simulink model "Adaptive_flux_observer_with_Rs_and_Rr_estimator"  (R2021a)
settings: Solver=FixedStepDiscrete  StartTime=0.0  StopTime=10.0  FixedStep=1e-5  RelTol=1e-3
undefined symbols (not defined in the file): DiscIntNeverNeededParam
settings Model: Creator=Mehra  LastModifiedBy=Mehra

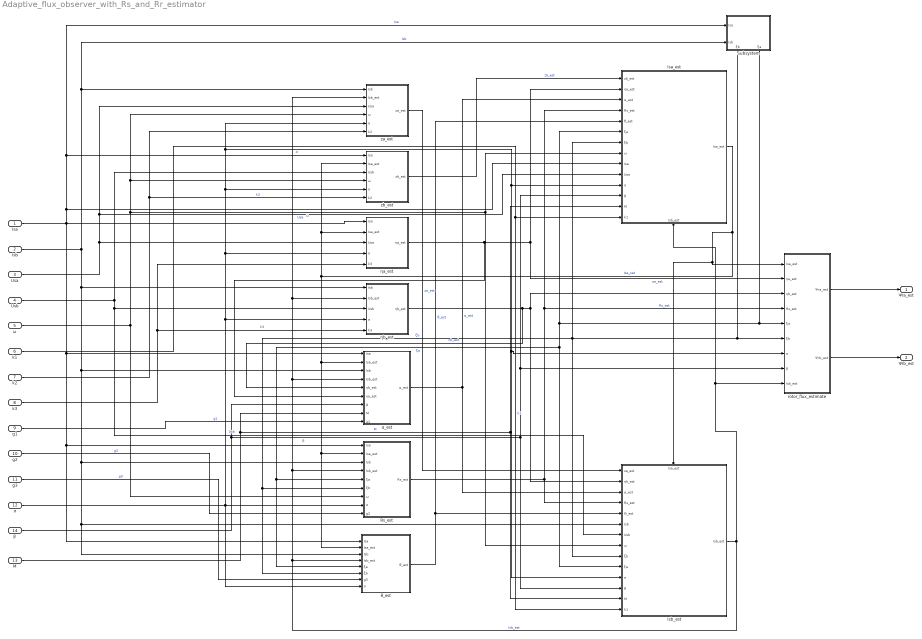
== system Adaptive_flux_observer_with_Rs_and_Rr_estimator ==
  Isa : Inport
  Isb : Inport  Port=2
  Usa : Inport  Port=3
  Usb : Inport  Port=4
  ω : Inport  Port=5
  k1 : Inport  Port=6
  k2 : Inport  Port=7
  k3 : Inport  Port=8
  g1 : Inport  Port=9
  g2 : Inport  Port=10
  g3 : Inport  Port=11
  σ : Inport  Port=12
  M : Inport  Port=13
  β : Inport  Port=14
  Isa_est : Subsystem
      settings: PortSchema="{\"entries\":[{\"content\":{\"sides\":[{\"content\":{\"connectorIds\":[\"In1\",\"In2\",\"In3\",\"In4\",\"In5\",\"In6\",\"In7\",\"In8\",\"In9\",\"In10\",\"In11\",\"In12\",\"In13\",\"In14\"]},\"type\":\"ConnectorPlacement.EquallySpacedRectSide\",\"uuid\":\"bb3cfb7f-73b8-4da7-b58a-4813aa7ccc08\"},{\"content\":{\"connectorIds\":[\"Out1\"],\"side\":\"RIGHT\"},\"type\":\"ConnectorPlacement.EquallySpacedRectSide\",\"uuid\":\"e2d64f82-074a-4c00-8fb2-34385227a041\"},{\"content\":{\"connectorIds\":[],\"side\":\"TOP\"},\"type\":\"ConnectorPlacement.EquallySpacedRectSide\",\"uuid\":\"410e12d1-af55-42b5-a1f1-21db609b2ad4\"},{\"content\":{\"connectorIds\":[\"In15\"],\"side\":\"BOTTOM\"},\"type\":\"ConnectorPlacement.EquallySpacedRectSide\",\"uuid\":\"b06c8fd3-df28-4480-a6c1-bf8451ef66bb\"}]},\"type\":\"ConnectorPlacement.EquallySpacedConnector\",\"uuid\":\"55afa802-9b43-40a4-afaf-7737924079c4\"}],\"packageUris\":[\"http://schema.mathworks.com/mf0/Connector/R2020b\"],\"version\":\"1.0\"}"
  Isb_est : Subsystem
      settings: PortSchema="{\"entries\":[{\"content\":{\"sides\":[{\"content\":{\"connectorIds\":[\"In1\",\"In2\",\"In3\",\"In4\",\"In5\",\"In6\",\"In7\",\"In8\",\"In9\",\"In10\",\"In11\",\"In12\",\"In13\",\"In14\"]},\"type\":\"ConnectorPlacement.EquallySpacedRectSide\",\"uuid\":\"bb3cfb7f-73b8-4da7-b58a-4813aa7ccc08\"},{\"content\":{\"connectorIds\":[\"Out1\"],\"side\":\"RIGHT\"},\"type\":\"ConnectorPlacement.EquallySpacedRectSide\",\"uuid\":\"e2d64f82-074a-4c00-8fb2-34385227a041\"},{\"content\":{\"connectorIds\":[\"In15\"],\"side\":\"TOP\"},\"type\":\"ConnectorPlacement.EquallySpacedRectSide\",\"uuid\":\"410e12d1-af55-42b5-a1f1-21db609b2ad4\"}]},\"type\":\"ConnectorPlacement.EquallySpacedConnector\",\"uuid\":\"55afa802-9b43-40a4-afaf-7737924079c4\"}],\"packageUris\":[\"http://schema.mathworks.com/mf0/Connector/R2020b\"],\"version\":\"1.0\"}"
  Rs_est : Subsystem
  Subsystem : Subsystem
      settings: PortSchema="{\"entries\":[{\"content\":{\"sides\":[{\"content\":{\"connectorIds\":[\"In1\",\"In2\"]},\"type\":\"ConnectorPlacement.EquallySpacedRectSide\",\"uuid\":\"a1d3c156-a5da-4fb5-b9de-670725af7275\"},{\"content\":{\"connectorIds\":[],\"side\":\"RIGHT\"},\"type\":\"ConnectorPlacement.EquallySpacedRectSide\",\"uuid\":\"3f754f1d-6fb2-4d8a-aa97-501505780465\"},{\"content\":{\"connectorIds\":[],\"side\":\"TOP\"},\"type\":\"ConnectorPlacement.EquallySpacedRectSide\",\"uuid\":\"d81724b2-7fa8-4949-b0ca-074282c9af04\"},{\"content\":{\"connectorIds\":[\"Out1\",\"Out2\"],\"side\":\"BOTTOM\"},\"type\":\"ConnectorPlacement.EquallySpacedRectSide\",\"uuid\":\"b126a6c9-2aef-47bb-af94-09140218a0dd\"}]},\"type\":\"ConnectorPlacement.EquallySpacedConnector\",\"uuid\":\"d3bdf017-892a-4548-9b2f-1467a9b3686f\"}],\"packageUris\":[\"http://schema.mathworks.com/mf0/Connector/R2020b\"],\"version\":\"1.0\"}"
  rotor_flux_estimate : Subsystem
  za_est : Subsystem
  zb_est : Subsystem
  α_est : Subsystem
  ηa_est : Subsystem
  ηb_est : Subsystem
  θ_est : Subsystem
  Ψra_est : Outport
  Ψrb_est : Outport  Port=2
  wires:
  Isa_est/1(Isa_est) -> zb_est/2(Isa_est), ηa_est/2(Isa_est), θ_est/2(Isa_est), Rs_est/2(Isa_est), α_est/2(Isa_est), Isb_est/15(Isa_est), rotor_flux_estimate/1(Isa_est)  "Isa_set"
  Isb_est/1(Isb_est) -> Isa_est/15(Isb_est), rotor_flux_estimate/9(Isb_est), za_est/2(Isb_est), ηb_est/2(Isb_est), α_est/4(Isb_est), Rs_est/4(Isb_est), θ_est/4(Isb_est)  "Isb_est"
  ηb_est/1(ηb_est) -> α_est/5(ηb_est), Isb_est/2(ηb_est), rotor_flux_estimate/3(ηb_est)  "ηb_est"
  ηa_est/1(ηa_est) -> α_est/6(ηa_est), Isa_est/2(ηa_est), rotor_flux_estimate/2(ηa_est)  "ηa_est"
  Subsystem/2(ξa) -> Isb_est/10(ξa), θ_est/5(ξa), Rs_est/5(ξa), Isa_est/6(ξa), rotor_flux_estimate/5(ξa)  "ξa"
  Subsystem/1(ξb) -> Isb_est/9(ξb), θ_est/6(ξb), Rs_est/6(ξb), Isa_est/7(ξb), rotor_flux_estimate/6(ξb)  "ξb"
  Rs_est/1(Rs_est) -> Isb_est/4(Rs_est), Isa_est/4(Rs_est), rotor_flux_estimate/4(Rs_est)  "Rs_est"
  zb_est/1(zb_est) -> Isa_est/1(zb_est)  "zb_est"
  α_est/1(α_est) -> Isb_est/3(α_est), Isa_est/3(α_est)  "α_est"
  θ_est/1(θ_est) -> Isb_est/5(Θ_est), Isa_est/5(θ_est)  "θ_est"
  za_est/1(za_est) -> Isb_est/1(za_est)  "za_est"
  Isb/1 -> θ_est/3(Isb), Isb_est/6(Isb), Rs_est/3(Isb), α_est/3(Isb), ηb_est/1(Isb), Subsystem/2(Isb), za_est/1(Isb)  "Isb"
  Usa/1 -> ηa_est/3(Usa), Isa_est/10(Usa), za_est/3(Usa)  "Usa"
  Isa/1 -> ηa_est/1(Isa), α_est/1(Isa), θ_est/1(Isa), Rs_est/1(Isa), Isa_est/9(Isa), Subsystem/1(Isa), zb_est/1(Isa)  "Isa"
  Usb/1 -> Isb_est/7(Usb), ηb_est/3(Usb), zb_est/3(Usb)  "Usb"
  ω/1 -> Rs_est/7(ω), Isa_est/8(ω), Isb_est/8(ω), zb_est/4(ω), za_est/4(ω)  "ω"
  g3/1 -> θ_est/7(g3)  "g3"
  g2/1 -> Rs_est/9(g2)  "g2"
  σ/1 -> θ_est/8(σ), Isa_est/11(σ), rotor_flux_estimate/7(σ), Isb_est/11(σ), za_est/5(σ), zb_est/5(σ), ηa_est/4(σ), ηb_est/4(σ), Rs_est/8(σ)  "σ"
  β/1 -> α_est/7(β), Isa_est/12(β), rotor_flux_estimate/8(β), Isb_est/12(β)  "β"
  M/1 -> Isa_est/13(M), Isb_est/13(M), α_est/8(M)  "M"
  k2/1 -> zb_est/6(k2), za_est/6(k2)  "k2"
  k3/1 -> ηb_est/5(k3), ηa_est/5(k3)  "k3"
  g1/1 -> α_est/9(g1)  "g1"
  k1/1 -> Isa_est/14(k1), Isb_est/14(k1)  "k1"
  rotor_flux_estimate/1(Ψra_est) -> Ψra_est/1
  rotor_flux_estimate/2(Ψrb_est) -> Ψrb_est/1

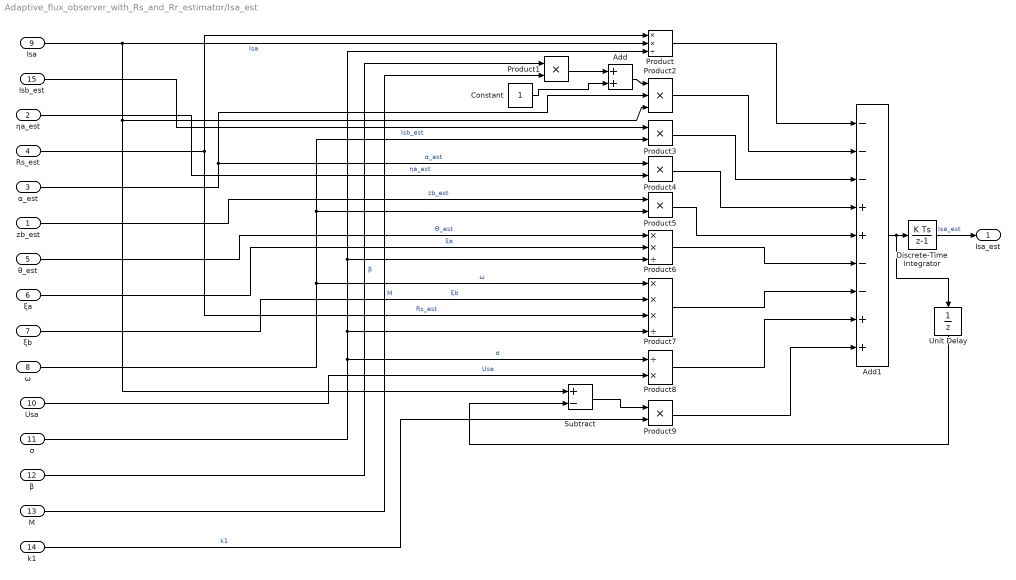
== system Adaptive_flux_observer_with_Rs_and_Rr_estimator/Isa_est ==
  zb_est : Inport
  ηa_est : Inport  Port=2
  α_est : Inport  Port=3
  Rs_est : Inport  Port=4
  θ_est : Inport  Port=5
  ξa : Inport  Port=6
  ξb : Inport  Port=7
  ω : Inport  Port=8
  Isa : Inport  Port=9
  Usa : Inport  Port=10
  σ : Inport  Port=11
  β : Inport  Port=12
  M : Inport  Port=13
  k1 : Inport  Port=14
  Isb_est : Inport  Port=15
  Add : Sum
  Add1 : Sum  Inputs=---++--++
  Constant : Constant
  Discrete-Time Integrator : DiscreteIntegrator  SampleTime=-1  ICPrevOutput=DiscIntNeverNeededParam  ICPrevScaledInput=DiscIntNeverNeededParam
  Product : Product  Inputs=**/
  Product{1,3..5,9} (5 alike) : Product
  Product2 : Product  Inputs=3
  Product6 : Product  Inputs=**/
  Product7 : Product  Inputs=***/
  Product8 : Product  Inputs=/*
  Subtract : Sum  Inputs=+-
  Unit Delay : UnitDelay  SampleTime=-1  HasFrameUpgradeWarning=on
  Isa_est : Outport
  wires:
  Rs_est/1 -> Product7/3, Product/1  "Rs_est"
  Isa/1 -> Product/2, Subtract/1, Product2/3  "Isa"
  σ/1 -> Product8/1, Product7/4, Product6/3, Product/3  "σ"
  Product1/1 -> Add/1
  Constant/1 -> Add/2
  β/1 -> Product1/1  "β"
  M/1 -> Product1/2  "M"
  Add/1 -> Product2/1
  α_est/1 -> Product4/1, Product2/2  "α_est"
  Isb_est/1 -> Product3/1  "Isb_est"
  ω/1 -> Product7/1, Product5/2, Product3/2  "ω"
  ηa_est/1 -> Product4/2  "ηa_est"
  zb_est/1 -> Product5/1  "zb_est"
  θ_est/1 -> Product6/1  "Θ_est"
  ξa/1 -> Product6/2  "ξa"
  ξb/1 -> Product7/2  "ξb"
  Usa/1 -> Product8/2  "Usa"
  Subtract/1 -> Product9/1
  k1/1 -> Product9/2  "k1"
  Discrete-Time Integrator/1 -> Isa_est/1  "Isa_est"
  Product/1 -> Add1/1
  Product2/1 -> Add1/2
  Product3/1 -> Add1/3
  Product4/1 -> Add1/4
  Product5/1 -> Add1/5
  Product6/1 -> Add1/6
  Product7/1 -> Add1/7
  Product8/1 -> Add1/8
  Product9/1 -> Add1/9
  Add1/1 -> Unit Delay/1, Discrete-Time Integrator/1
  Unit Delay/1 -> Subtract/2

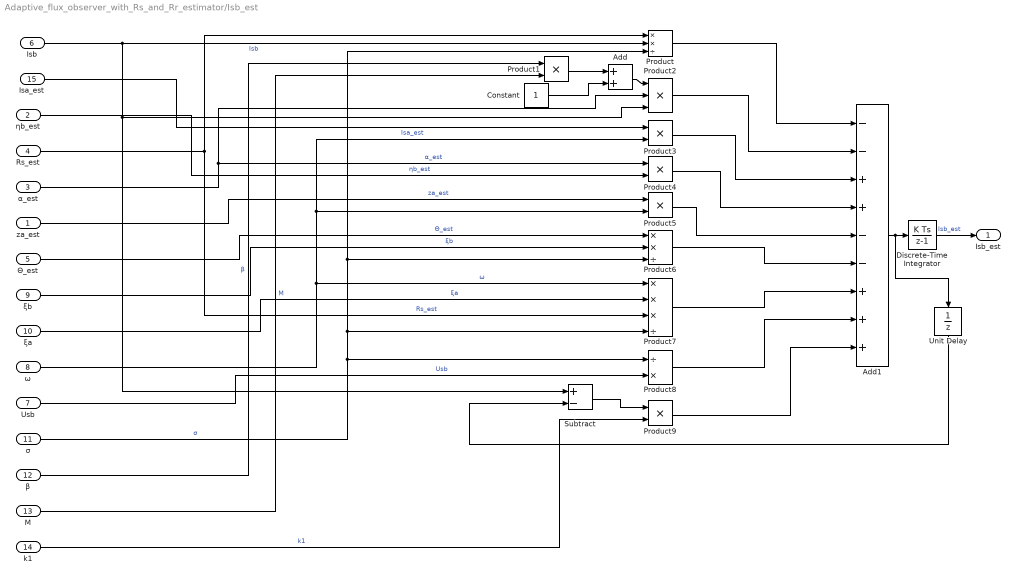
== system Adaptive_flux_observer_with_Rs_and_Rr_estimator/Isb_est ==
  za_est : Inport
  ηb_est : Inport  Port=2
  α_est : Inport  Port=3
  Rs_est : Inport  Port=4
  Θ_est : Inport  Port=5
  Isb : Inport  Port=6
  Usb : Inport  Port=7
  ω : Inport  Port=8
  ξb : Inport  Port=9
  ξa : Inport  Port=10
  σ : Inport  Port=11
  β : Inport  Port=12
  M : Inport  Port=13
  k1 : Inport  Port=14
  Isa_est : Inport  Port=15
  Add : Sum
  Add1 : Sum  Inputs=--++--+++
  Constant : Constant
  Discrete-Time Integrator : DiscreteIntegrator  SampleTime=-1  ICPrevOutput=DiscIntNeverNeededParam  ICPrevScaledInput=DiscIntNeverNeededParam
  Product : Product  Inputs=**/
  Product{1,3..5,9} (5 alike) : Product
  Product2 : Product  Inputs=3
  Product6 : Product  Inputs=**/
  Product7 : Product  Inputs=***/
  Product8 : Product  Inputs=/*
  Subtract : Sum  Inputs=+-
  Unit Delay : UnitDelay  SampleTime=-1  HasFrameUpgradeWarning=on
  Isb_est : Outport
  wires:
  Rs_est/1 -> Product7/3, Product/1  "Rs_est"
  Isb/1 -> Product/2, Subtract/1, Product2/3  "Isb"
  σ/1 -> Product8/1, Product7/4, Product6/3, Product/3  "σ"
  Product1/1 -> Add/1
  Constant/1 -> Add/2
  β/1 -> Product1/1  "β"
  M/1 -> Product1/2  "M"
  Add/1 -> Product2/1
  α_est/1 -> Product4/1, Product2/2  "α_est"
  Isa_est/1 -> Product3/1  "Isa_est"
  ω/1 -> Product7/1, Product5/2, Product3/2  "ω"
  ηb_est/1 -> Product4/2  "ηb_est"
  za_est/1 -> Product5/1  "za_est"
  Θ_est/1 -> Product6/1  "Θ_est"
  ξb/1 -> Product6/2  "ξb"
  ξa/1 -> Product7/2  "ξa"
  Usb/1 -> Product8/2  "Usb"
  Subtract/1 -> Product9/1
  k1/1 -> Product9/2  "k1"
  Discrete-Time Integrator/1 -> Isb_est/1  "Isb_est"
  Product/1 -> Add1/1
  Product2/1 -> Add1/2
  Product3/1 -> Add1/3
  Product4/1 -> Add1/4
  Product5/1 -> Add1/5
  Product6/1 -> Add1/6
  Product7/1 -> Add1/7
  Product8/1 -> Add1/8
  Product9/1 -> Add1/9
  Add1/1 -> Unit Delay/1, Discrete-Time Integrator/1
  Unit Delay/1 -> Subtract/2

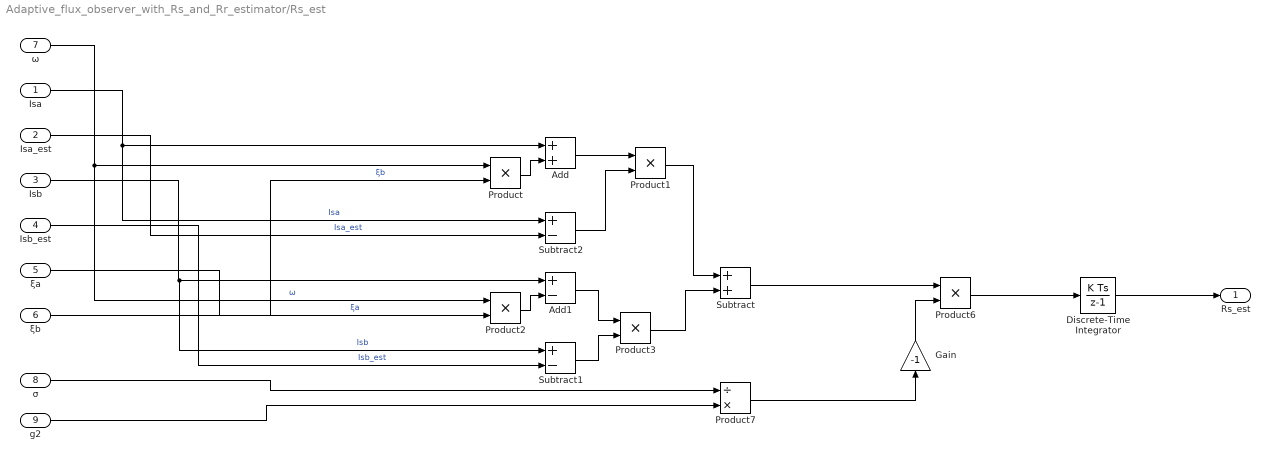
== system Adaptive_flux_observer_with_Rs_and_Rr_estimator/Rs_est ==
  Isa : Inport
  Isa_est : Inport  Port=2
  Isb : Inport  Port=3
  Isb_est : Inport  Port=4
  ξa : Inport  Port=5
  ξb : Inport  Port=6
  ω : Inport  Port=7
  σ : Inport  Port=8
  g2 : Inport  Port=9
  Add : Sum
  Add1 : Sum  Inputs=+-
  Discrete-Time Integrator : DiscreteIntegrator  SampleTime=-1  ICPrevOutput=DiscIntNeverNeededParam  ICPrevScaledInput=DiscIntNeverNeededParam
  Gain : Gain  Gain=-1
  Product{,1..3,6} (5 alike) : Product
  Product7 : Product  Inputs=/*
  Subtract : Sum
  Subtract1 : Sum  Inputs=+-
  Subtract2 : Sum  Inputs=+-
  Rs_est : Outport
  wires:
  Add/1 -> Product1/1
  Product1/1 -> Subtract/1
  Subtract/1 -> Product6/1
  g2/1 -> Product7/2
  Gain/1 -> Product6/2
  Product6/1 -> Discrete-Time Integrator/1
  Discrete-Time Integrator/1 -> Rs_est/1
  Product7/1 -> Gain/1
  σ/1 -> Product7/1
  Product/1 -> Add/2
  Subtract2/1 -> Product1/2
  Product3/1 -> Subtract/2
  Product2/1 -> Add1/2
  Add1/1 -> Product3/1
  Subtract1/1 -> Product3/2
  Isa/1 -> Subtract2/1, Add/1  "Isa"
  ω/1 -> Product2/1, Product/1  "ω"
  ξb/1 -> Product/2  "ξb"
  Isa_est/1 -> Subtract2/2  "Isa_est"
  Isb/1 -> Subtract1/1, Add1/1  "Isb"
  ξa/1 -> Product2/2  "ξa"
  Isb_est/1 -> Subtract1/2  "Isb_est"

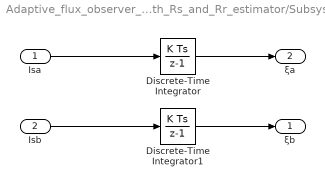
== system Adaptive_flux_observer_with_Rs_and_Rr_estimator/Subsystem ==
  Isa : Inport
  Isb : Inport  Port=2
  Discrete-Time Integrator : DiscreteIntegrator  SampleTime=-1  ICPrevOutput=DiscIntNeverNeededParam  ICPrevScaledInput=DiscIntNeverNeededParam
  Discrete-Time Integrator1 : DiscreteIntegrator  SampleTime=-1  ICPrevOutput=DiscIntNeverNeededParam  ICPrevScaledInput=DiscIntNeverNeededParam
  ξb : Outport
  ξa : Outport  Port=2
  wires:
  Isa/1 -> Discrete-Time Integrator/1
  Discrete-Time Integrator/1 -> ξa/1
  Isb/1 -> Discrete-Time Integrator1/1
  Discrete-Time Integrator1/1 -> ξb/1

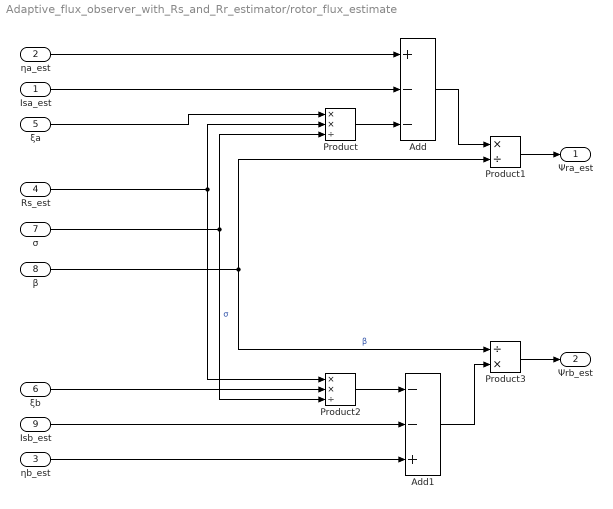
== system Adaptive_flux_observer_with_Rs_and_Rr_estimator/rotor_flux_estimate ==
  Isa_est : Inport
  ηa_est : Inport  Port=2
  ηb_est : Inport  Port=3
  Rs_est : Inport  Port=4
  ξa : Inport  Port=5
  ξb : Inport  Port=6
  σ : Inport  Port=7
  β : Inport  Port=8
  Isb_est : Inport  Port=9
  Add : Sum  Inputs=+--
  Add1 : Sum  Inputs=--+
  Product : Product  Inputs=**/
  Product1 : Product  Inputs=*/
  Product2 : Product  Inputs=**/
  Product3 : Product  Inputs=/*
  Ψra_est : Outport
  Ψrb_est : Outport  Port=2
  wires:
  ηa_est/1 -> Add/1
  Isa_est/1 -> Add/2
  Product/1 -> Add/3
  ξa/1 -> Product/1
  Rs_est/1 -> Product2/1, Product/2
  σ/1 -> Product2/3, Product/3  "σ"
  Add/1 -> Product1/1
  β/1 -> Product3/1, Product1/2  "β"
  Product1/1 -> Ψra_est/1
  Product2/1 -> Add1/1
  ξb/1 -> Product2/2
  Isb_est/1 -> Add1/2
  ηb_est/1 -> Add1/3
  Add1/1 -> Product3/2
  Product3/1 -> Ψrb_est/1

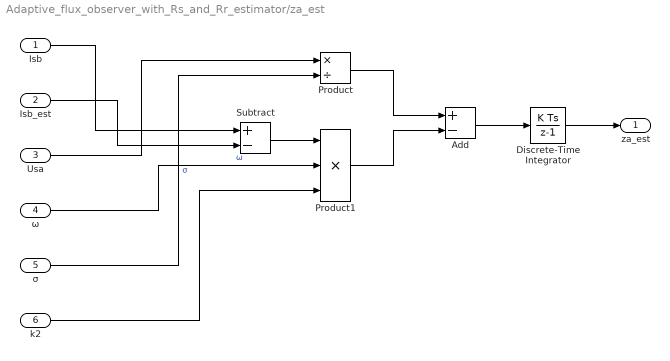
== system Adaptive_flux_observer_with_Rs_and_Rr_estimator/za_est ==
  Isb : Inport
  Isb_est : Inport  Port=2
  Usa : Inport  Port=3
  ω : Inport  Port=4
  σ : Inport  Port=5
  k2 : Inport  Port=6
  Add : Sum  Inputs=+-
  Discrete-Time Integrator : DiscreteIntegrator  SampleTime=-1  ICPrevOutput=DiscIntNeverNeededParam  ICPrevScaledInput=DiscIntNeverNeededParam
  Product : Product  Inputs=*/
  Product1 : Product  Inputs=3
  Subtract : Sum  Inputs=+-
  za_est : Outport
  wires:
  Usa/1 -> Product/1
  σ/1 -> Product/2  "σ"
  k2/1 -> Product1/3
  ω/1 -> Product1/2  "ω"
  Subtract/1 -> Product1/1
  Isb/1 -> Subtract/1
  Isb_est/1 -> Subtract/2
  Product/1 -> Add/1
  Product1/1 -> Add/2
  Add/1 -> Discrete-Time Integrator/1
  Discrete-Time Integrator/1 -> za_est/1

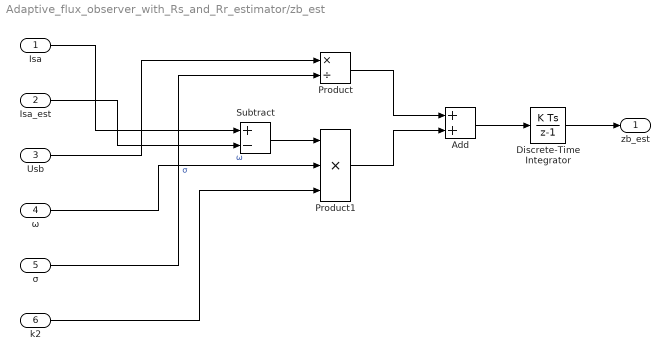
== system Adaptive_flux_observer_with_Rs_and_Rr_estimator/zb_est ==
  Isa : Inport
  Isa_est : Inport  Port=2
  Usb : Inport  Port=3
  ω : Inport  Port=4
  σ : Inport  Port=5
  k2 : Inport  Port=6
  Add : Sum
  Discrete-Time Integrator : DiscreteIntegrator  SampleTime=-1  ICPrevOutput=DiscIntNeverNeededParam  ICPrevScaledInput=DiscIntNeverNeededParam
  Product : Product  Inputs=*/
  Product1 : Product  Inputs=3
  Subtract : Sum  Inputs=+-
  zb_est : Outport
  wires:
  Usb/1 -> Product/1
  σ/1 -> Product/2  "σ"
  k2/1 -> Product1/3
  ω/1 -> Product1/2  "ω"
  Subtract/1 -> Product1/1
  Isa/1 -> Subtract/1
  Isa_est/1 -> Subtract/2
  Product/1 -> Add/1
  Product1/1 -> Add/2
  Add/1 -> Discrete-Time Integrator/1
  Discrete-Time Integrator/1 -> zb_est/1

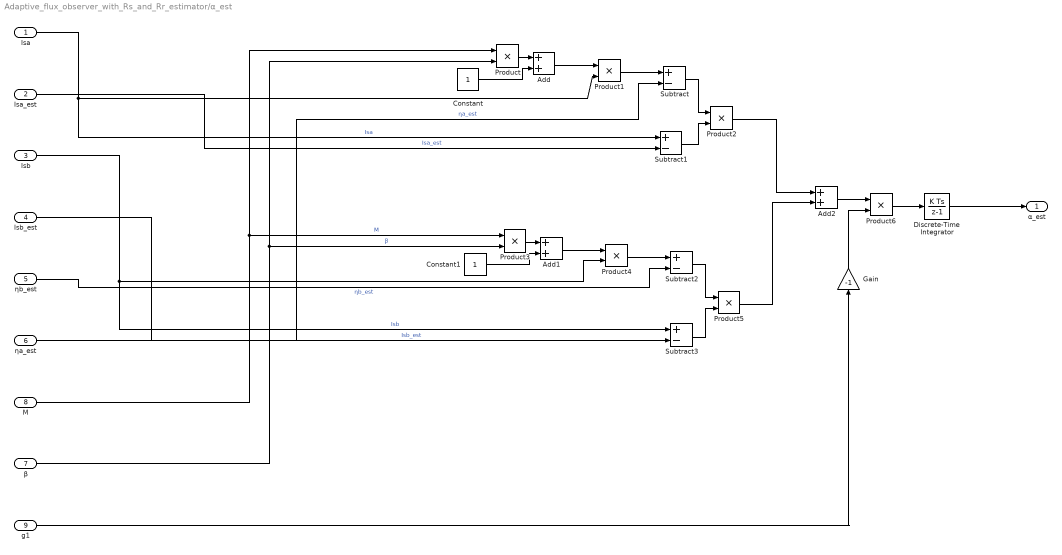
== system Adaptive_flux_observer_with_Rs_and_Rr_estimator/α_est ==
  Isa : Inport
  Isa_est : Inport  Port=2
  Isb : Inport  Port=3
  Isb_est : Inport  Port=4
  ηb_est : Inport  Port=5
  ηa_est : Inport  Port=6
  β : Inport  Port=7
  M : Inport  Port=8
  g1 : Inport  Port=9
  Add : Sum
  Add1 : Sum
  Add2 : Sum
  Constant : Constant
  Constant1 : Constant
  Discrete-Time Integrator : DiscreteIntegrator  SampleTime=-1  ICPrevOutput=DiscIntNeverNeededParam  ICPrevScaledInput=DiscIntNeverNeededParam
  Gain : Gain  Gain=-1
  Product{,1..6} (7 alike) : Product
  Subtract{,1..3} (4 alike) : Sum  Inputs=+-
  α_est : Outport
  wires:
  Product5/1 -> Add2/2
  Isa/1 -> Subtract1/1, Product1/2  "Isa"
  Product2/1 -> Add2/1
  Subtract/1 -> Product2/1
  Isa_est/1 -> Subtract1/2  "Isa_est"
  ηb_est/1 -> Subtract2/2  "ηb_est"
  Product4/1 -> Subtract2/1
  M/1 -> Product3/1, Product/1  "M"
  Product/1 -> Add/1
  Subtract3/1 -> Product5/2
  β/1 -> Product/2, Product3/2  "β"
  ηa_est/1 -> Subtract/2  "ηa_est"
  Constant1/1 -> Add1/2
  Subtract1/1 -> Product2/2
  Product3/1 -> Add1/1
  Add1/1 -> Product4/1
  Isb/1 -> Product4/2, Subtract3/1  "Isb"
  Subtract2/1 -> Product5/1
  Add/1 -> Product1/1
  Isb_est/1 -> Subtract3/2  "Isb_est"
  Constant/1 -> Add/2
  Product1/1 -> Subtract/1
  Add2/1 -> Product6/1
  g1/1 -> Gain/1
  Gain/1 -> Product6/2
  Product6/1 -> Discrete-Time Integrator/1
  Discrete-Time Integrator/1 -> α_est/1

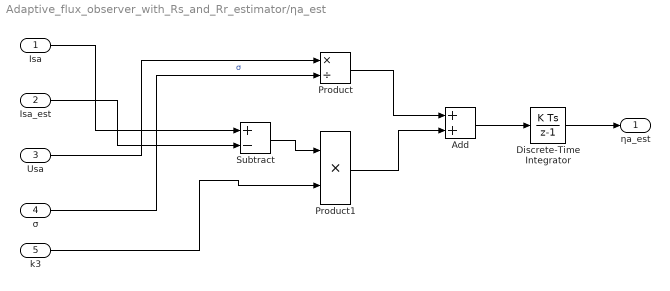
== system Adaptive_flux_observer_with_Rs_and_Rr_estimator/ηa_est ==
  Isa : Inport
  Isa_est : Inport  Port=2
  Usa : Inport  Port=3
  σ : Inport  Port=4
  k3 : Inport  Port=5
  Add : Sum
  Discrete-Time Integrator : DiscreteIntegrator  SampleTime=-1  ICPrevOutput=DiscIntNeverNeededParam  ICPrevScaledInput=DiscIntNeverNeededParam
  Product : Product  Inputs=*/
  Product1 : Product
  Subtract : Sum  Inputs=+-
  ηa_est : Outport
  wires:
  Usa/1 -> Product/1
  σ/1 -> Product/2  "σ"
  k3/1 -> Product1/2
  Subtract/1 -> Product1/1
  Isa/1 -> Subtract/1
  Isa_est/1 -> Subtract/2
  Product/1 -> Add/1
  Product1/1 -> Add/2
  Add/1 -> Discrete-Time Integrator/1
  Discrete-Time Integrator/1 -> ηa_est/1

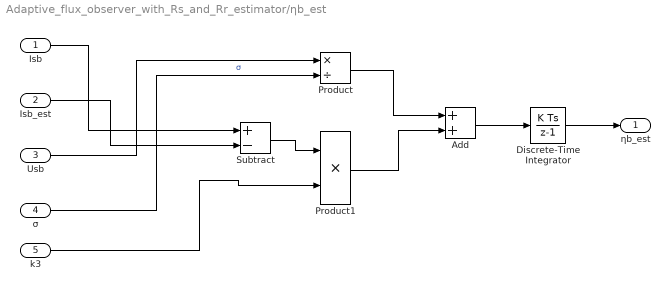
== system Adaptive_flux_observer_with_Rs_and_Rr_estimator/ηb_est ==
  Isb : Inport
  Isb_est : Inport  Port=2
  Usb : Inport  Port=3
  σ : Inport  Port=4
  k3 : Inport  Port=5
  Add : Sum
  Discrete-Time Integrator : DiscreteIntegrator  SampleTime=-1  ICPrevOutput=DiscIntNeverNeededParam  ICPrevScaledInput=DiscIntNeverNeededParam
  Product : Product  Inputs=*/
  Product1 : Product
  Subtract : Sum  Inputs=+-
  ηb_est : Outport
  wires:
  Usb/1 -> Product/1
  σ/1 -> Product/2  "σ"
  k3/1 -> Product1/2
  Subtract/1 -> Product1/1
  Isb/1 -> Subtract/1
  Isb_est/1 -> Subtract/2
  Product/1 -> Add/1
  Product1/1 -> Add/2
  Add/1 -> Discrete-Time Integrator/1
  Discrete-Time Integrator/1 -> ηb_est/1

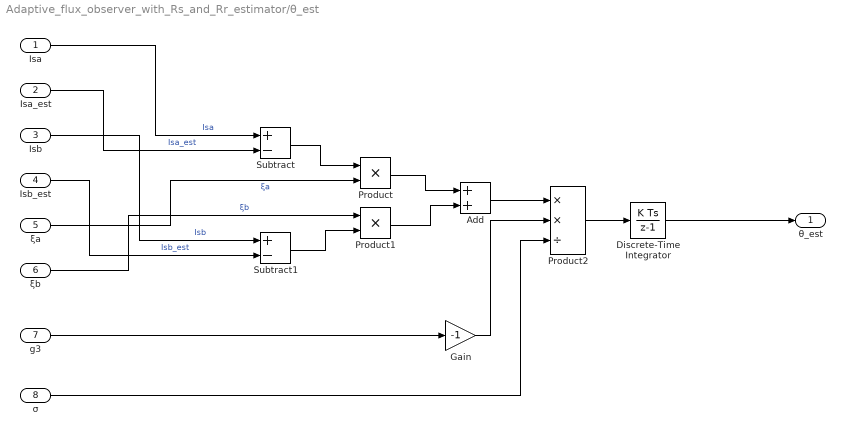
== system Adaptive_flux_observer_with_Rs_and_Rr_estimator/θ_est ==
  Isa : Inport
  Isa_est : Inport  Port=2
  Isb : Inport  Port=3
  Isb_est : Inport  Port=4
  ξa : Inport  Port=5
  ξb : Inport  Port=6
  g3 : Inport  Port=7
  σ : Inport  Port=8
  Add : Sum
  Discrete-Time Integrator : DiscreteIntegrator  SampleTime=-1  ICPrevOutput=DiscIntNeverNeededParam  ICPrevScaledInput=DiscIntNeverNeededParam
  Gain : Gain  Gain=-1
  Product : Product
  Product1 : Product
  Product2 : Product  Inputs=**/
  Subtract : Sum  Inputs=+-
  Subtract1 : Sum  Inputs=+-
  θ_est : Outport
  wires:
  Product/1 -> Add/1
  Product1/1 -> Add/2
  Subtract/1 -> Product/1
  Subtract1/1 -> Product1/2
  Add/1 -> Product2/1
  Product2/1 -> Discrete-Time Integrator/1
  Discrete-Time Integrator/1 -> θ_est/1
  g3/1 -> Gain/1
  σ/1 -> Product2/3
  Gain/1 -> Product2/2
  Isa/1 -> Subtract/1  "Isa"
  Isa_est/1 -> Subtract/2  "Isa_est"
  ξa/1 -> Product/2  "ξa"
  ξb/1 -> Product1/1  "ξb"
  Isb/1 -> Subtract1/1  "Isb"
  Isb_est/1 -> Subtract1/2  "Isb_est"
